simulink model "cCodeTester"  (R2024b)
settings: Solver=FixedStepAuto  StartTime=0.0  StopTime=10  FixedStep=1e-3  RelTol=1e-3
model workspace (MAT data in the model file):
  alpha = 0.5
undefined symbols (not defined in the file): gaussian, SampleTime
libraries: simulink x7, slpidlib x1
settings Model: Creator=karadeli  LastModifiedBy=karadeli
settings OptimizationCC: BlockReduction=off
settings SFSimCC: SimCustomHeaderCode=|
  | #include "myMalloc.h"
  | #include "pid.h"
  | #include "filter.h"
settings SFSimCC: SimUserSources=|
  | filter.c
  | myMalloc.c
  | pid.c
settings RTWCC: GPUComputeCapability=3.5

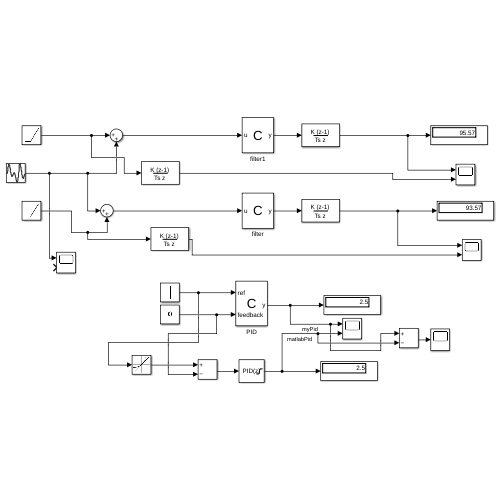
[thumbnail: Simulink's stored preview of the top-level diagram]
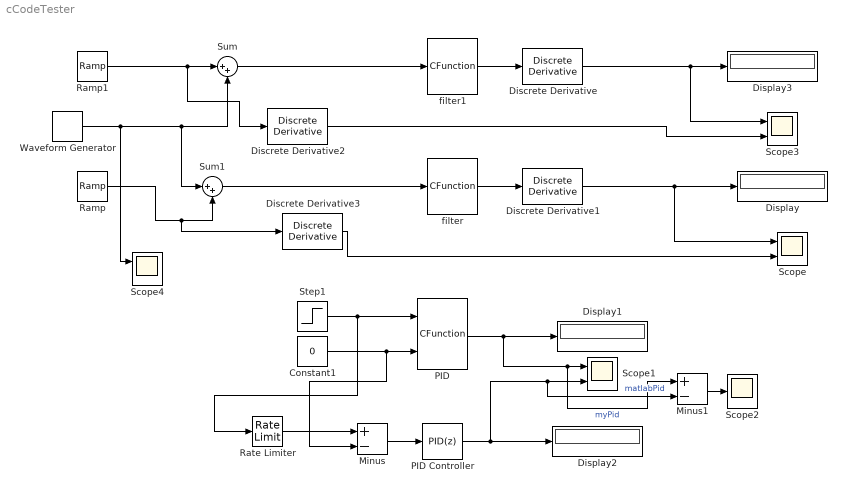
== system cCodeTester ==
  Constant1 : Constant  Value=0
  Discrete Derivative{,1..3} (4 alike) : simulink/Discrete/Discrete Derivative  gainval=1.0  ICPrevScaledInput=0.0  OutMin=[]  OutMax=[]  OutDataType=fixdt(1, 16)  OutScaling=2^-10  DoSatur=off
  Display{,1..3} (4 alike) : Display
  Minus : Sum  Inputs=+-
  Minus1 : Sum  Inputs=+-
  PID : CFunction  OutputCode=|  StartCode=|  GenerateCodeAsIs=off  CodegenOutputCode=|  CodegenStartCode=|  SampleTime=SampleTime  CustomCodeSettingLocation=ModelConfigurationParameters  kP=2  kI=1  kD=0.1  kFF=0  dT=1e-3  rateLimMax=1  saturationMax=5  integralSaturationMax=0.5  integralActiveBandMax=1000  SampleTime=1e-3
      OutputCode=|
      | pid_controller_s *myPid = pid;
      | ref_int = ref;
      | feedback_int = feedback;
      | pid_controller_iterate(myPid);
      | y= myPid->y;
      StartCode=|
      | params = myMalloc(sizeof(pid_parameters_s));
      | pid = myMalloc(sizeof(pid_controller_s));
      | 
      | pid_parameters_s *params_p = params;
      | pid_controller_s *pid_p = pid;
      | 
      | params_p->kP = kP;
      | params_p->kI = kI;
      | params_p->kD = kD;
      | params_p->kFF = kFF;
      | params_p->dT = dT;
      | params_p->rateLimitMax = rateLimMax;
      | params_p->rateLimitMin = -rateLimMax;
      | params_p->saturationMax = saturationMax;
      | params_p->saturationMin = - saturationMax;
      | params_p->integralSaturationMax = integralSaturationMax;
      | params_p->integralSaturationMin = -integralSaturationMax;
      | params_p->integralActiveBandMax = integralActiveBandMax;
      | params_p->integralActiveBandMin = -integralActiveBandMax;
      | 
      | ref_int = 0.0;
      | feedback_int = 0.0;
      | 
      | pid_controller_init(pid_p,params_p,&ref_int, &feedback_int);
      CodegenOutputCode=|
      | pid_controller_s *myPid = pid;
      | ref_int = ref;
      | feedback_int = feedback;
      | pid_controller_iterate(myPid);
      | y= myPid->y;
      CodegenStartCode=|
      | params = myMalloc(sizeof(pid_parameters_s));
      | pid = myMalloc(sizeof(pid_controller_s));
      | 
      | pid_parameters_s *params_p = params;
      | pid_controller_s *pid_p = pid;
      | 
      | params_p->kP = kP;
      | params_p->kI = kI;
      | params_p->kD = kD;
      | params_p->kFF = kFF;
      | params_p->dT = dT;
      | params_p->rateLimitMax = rateLimMax;
      | params_p->rateLimitMin = -rateLimMax;
      | params_p->saturationMax = saturationMax;
      | params_p->saturationMin = - saturationMax;
      | params_p->integralSaturationMax = integralSaturationMax;
      | params_p->integralSaturationMin = -integralSaturationMax;
      | params_p->integralActiveBandMax = integralActiveBandMax;
      | params_p->integralActiveBandMin = -integralActiveBandMax;
      | 
      | ref_int = 0.0;
      | feedback_int = 0.0;
      | 
      | pid_controller_init(pid_p,params_p,&ref_int, &feedback_int);
  PID Controller : slpidlib/PID Controller  Controller=PID  Form=Parallel  TimeDomain=Discrete-time  UseExternalTs=off  SampleTime=1e-3  IntegratorMethod=Forward Euler  FilterMethod=Forward Euler  ControllerParametersSource=internal  P=2  I=1  UseKiTs=off  D=0.1  UseExternalDerivativeSource=off  N=0  UseFilter=off  TunerSelectOption=Transfer Function Based (PID Tuner App)  InitialConditionSource=internal  InitialConditionForIntegrator=0  InitialConditionForFilter=0  DifferentiatorICPrevScaledInput=0  ExternalReset=none  TrackingMode=off  Kt=1  LimitOutput=on  SatLimitsSource=internal  UpperSaturationLimit=5  LowerSaturationLimit=-5  LinearizeAsGain=on  AntiWindupMode=none  Kb=1  LimitIntegrator=on  UpperIntegratorSaturationLimit=0.5  LowerIntegratorSaturationLimit=-0.5  POutMin=[]  POutMax=[]  IOutMin=[]  IOutMax=[]  DOutMin=[]  DOutMax=[]  NOutMin=[]  NOutMax=[]  SumOutMin=[]  SumOutMax=[]  SaturationOutMin=[]  SaturationOutMax=[]  PParamMin=[]  PParamMax=[]  IParamMin=[]  IParamMax=[]  DParamMin=[]  DParamMax=[]  NParamMin=[]  NParamMax=[]  KbParamMin=[]  KbParamMax=[]  KtParamMin=[]  KtParamMax=[]  KbOutMin=[]  KbOutMax=[]  KtOutMin=[]  KtOutMax=[]  IntegratorOutMin=[]  IntegratorOutMax=[]  FilterOutMin=[]  FilterOutMax=[]  SumI1OutMin=[]  SumI1OutMax=[]  SumI2OutMin=[]  SumI2OutMax=[]  SumI3OutMin=[]  SumI3OutMax=[]  SumI4OutMin=[]  SumI4OutMax=[]  SumDOutMin=[]  SumDOutMax=[]  DifferentiatorOutMin=[]  DifferentiatorOutMax=[]  FilterDiffOutCoefMin=[]  FilterDiffOutCoefMax=[]  ReciprocalOutMin=[]  ReciprocalOutMax=[]  SumDenOutMin=[]  SumDenOutMax=[]  SumNumOutMin=[]  SumNumOutMax=[]  DivideOutMin=[]  DivideOutMax=[]  UdiffTsProdOutMin=[]  UdiffTsProdOutMax=[]  NTsProdOutMin=[]  NTsProdOutMax=[]  UintegralTsProdOutMin=[]  UintegralTsProdOutMax=[]  UngainTsProdOutMin=[]  UngainTsProdOutMax=[]  ClampingZeroOutDataTypeStr=Inherit: Inherit via back propagation  ClampingZeroOutMin=[]  ClampingZeroOutMax=[]  FilterDenConstantOutDataTypeStr=Inherit: Inherit via back propagation  FilterDenConstantOutMin=[]  FilterDenConstantOutMax=[]  PCopyOutDataTypeStr=Inherit: Inherit via back propagation  PCopyOutMin=[]  PCopyOutMax=[]  NCopyOutDataTypeStr=Inherit: Inherit via back propagation  NCopyOutMin=[]  NCopyOutMax=[]  IntegratorContinuousStateAttributes=''  IntegratorStateMustResolveToSignalObject=off  IntegratorRTWStateStorageClass=Auto  FilterContinuousStateAttributes=''  FilterStateMustResolveToSignalObject=off  FilterRTWStateStorageClass=Auto  ParallelPVariant=InternalParameters  IdealPVariant=Disabled  IVariant=InternalParameters  DVariant=InternalParameters  IntegratorVariant=Discrete  SatVariant=Enabled  AWVariant=Passthrough  PCopyVariant=Disabled  TRVariant=Disabled  FdbkBlocksVariant=Forward  IdealPFdbkVariant=Disabled  SatFdbkVariant=Disabled  DerivativeFilterVariant=Differentiator  NVariant=Passthrough  NCopyVariant=Disabled_SignalSpec  FilterICVariant=InternalICsDifferentiator  IntegratorICVariant=InternalICs  ExternalResetVariant=Disabled  TRSumVariant=Passthrough  SumFdbkVariant=Disabled  SumVariant=Sum_PID  TsampFilterVariant=InternalTs  TsampNgainVariant=Passthrough  TsampIntegralVariant=Disabled_SignalSpec  ExternalSaturationOutDataTypeStr=Inherit: Same as second input  DerivativeSourceVariant=ErrorSignal  PreIntVariant=InternalPreInt
  Ramp : simulink/Sources/Ramp  slope=1  start=0  InitialOutput=0
  Ramp1 : simulink/Sources/Ramp  slope=3  start=0  InitialOutput=0
  Rate Limiter : RateLimiter  SampleTimeMode=inherited
  Scope{,1,3..4} (4 alike) : Scope  NumInputPorts=2
  Scope2 : Scope
  Step1 : Step  SampleTime=0
  Sum : Sum  Inputs=|++
  Sum1 : Sum  Inputs=|++
  Waveform Generator : simulink/Sources/Waveform Generator  OutMin=[]  OutMax=[]  OutDataTypeStr=double  SelectedSignal=1  Signals=gaussian(0,0.5,31693131)  BlockNames=MultiportSwitch_975190b9ceca4a0  SampleTime=1e-3
  filter : CFunction  OutputCode=|  StartCode=|  GenerateCodeAsIs=off  CodegenOutputCode=|  CodegenStartCode=|  SampleTime=SampleTime  CustomCodeSettingLocation=ModelConfigurationParameters  alpha=0.1  SampleTime=1e-3
      OutputCode=|
      | ema_filter_s *myFilter = pointer;
      | u_internal = u;
      | ema_filter_iter(myFilter);
      | 
      | y = myFilter->y;
      StartCode=|
      | pointer = myMalloc(sizeof(ema_filter_s));
      | u_internal = 0.0;
      | 
      | ema_filter_init(pointer, &u_internal, alpha);
      CodegenOutputCode=|
      | ema_filter_s *myFilter = pointer;
      | u_internal = u;
      | ema_filter_iter(myFilter);
      | 
      | y = myFilter->y;
      CodegenStartCode=|
      | pointer = myMalloc(sizeof(ema_filter_s));
      | u_internal = 0.0;
      | 
      | ema_filter_init(pointer, &u_internal, alpha);
  filter1 : CFunction  OutputCode=|  StartCode=|  GenerateCodeAsIs=off  CodegenOutputCode=|  CodegenStartCode=|  SampleTime=SampleTime  CustomCodeSettingLocation=ModelConfigurationParameters  alpha=0.1  SampleTime=1e-3
      OutputCode=|
      | ema_filter_s *myFilter = pointer;
      | u_internal = u;
      | ema_filter_iter(myFilter);
      | 
      | y = myFilter->y;
      StartCode=|
      | pointer = myMalloc(sizeof(ema_filter_s));
      | u_internal = 0.0;
      | 
      | ema_filter_init(pointer, &u_internal, alpha);
      CodegenOutputCode=|
      | ema_filter_s *myFilter = pointer;
      | u_internal = u;
      | ema_filter_iter(myFilter);
      | 
      | y = myFilter->y;
      CodegenStartCode=|
      | pointer = myMalloc(sizeof(ema_filter_s));
      | u_internal = 0.0;
      | 
      | ema_filter_init(pointer, &u_internal, alpha);
  wires:
  Sum1/1 -> filter/1
  filter/1 -> Discrete Derivative1/1
  Step1/1 -> Rate Limiter/1, PID/1
  Constant1/1 -> Minus/2, PID/2
  Minus/1 -> PID Controller/1
  PID Controller/1 -> Minus1/2, Scope1/2, Display2/1  "matlabPid"
  PID/1 -> Minus1/1, Scope1/1, Display1/1  "myPid"
  Minus1/1 -> Scope2/1
  Rate Limiter/1 -> Minus/1
  Sum/1 -> filter1/1
  Ramp1/1 -> Discrete Derivative2/1, Sum/1
  Waveform Generator/1 -> Scope4/1, Sum1/1, Sum/2
  Ramp/1 -> Discrete Derivative3/1, Sum1/2
  filter1/1 -> Discrete Derivative/1
  Discrete Derivative/1 -> Scope3/1, Display3/1
  Discrete Derivative1/1 -> Scope/1, Display/1
  Discrete Derivative2/1 -> Scope3/2
  Discrete Derivative3/1 -> Scope/2
